simulink model "sphere_6SUR_mech"  (R2017a)
settings: Solver=FixedStepAuto  StartTime=0.0  StopTime=100  FixedStep=0.001  RelTol=1e-2  EnableMultiTasking=on
undefined symbols (not defined in the file): m, rad, s
libraries: mblibv1 x69, simulink x3, instrumentlib x1
(part 2 of 2)

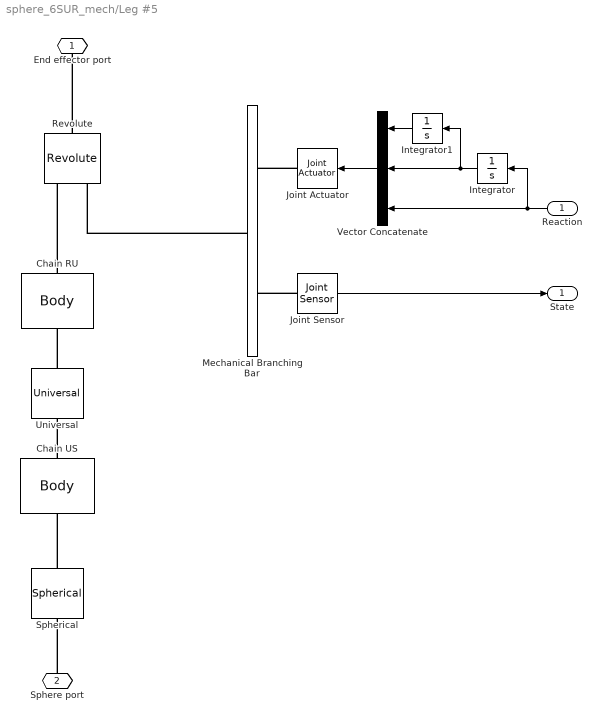
== system sphere_6SUR_mech/Leg #5 ==
  Reaction : Inport
  Chain RU : mblibv1/Bodies/Body  LConnTagsString=CS1  RConnTagsString=CS2  UpdateFromCAD=off  DialogClass=MechanicalBodyBlock  Mass=ru_mass  MassUnits=kg  InertiaUnits=kg*m^2  Inertia=zeros(3)  Shape=Cylinder  ShapeDims=[1 1]  ShapeUnits=m  ShapeUse=false  Density=1  DensityUnits=kg/m^3  DensityUse=false  GraphicsMode=CONVHULL  BodyColorSelMode=COLORPALETTE  BodyColor=[0 1 0]  AttachedToCS=CG  CG=Left$CG$(u_coord+r_coord)/2$World$World$m$[0 0 0]$Euler X-Y-Z$deg$World$false$none  WorkingFrames=Left$CS1$u_coord$World$World$m$[0 0 0]$Euler X-Y-Z$deg$World$true$none#Right$CS2$r_coord$World$World$m$[0 0 0]$Euler X-Y-Z$deg$World$true$none  CGPos=(u_coord+r_coord)/2  CGRot=[0 0 0]  CS0Pos=[]  CS0Rot=[]  CS1Pos=u_coord  CS1Rot=[0 0 0]  CS2Pos=r_coord  CS2Rot=[0 0 0]  CS3Pos=[]  CS3Rot=[]  CS4Pos=[]  CS4Rot=[]  CS5Pos=[]  CS5Rot=[]  CS6Pos=[]  CS6Rot=[]  CS7Pos=[]  CS7Rot=[]  CS8Pos=[]  CS8Rot=[]  CS9Pos=[]  CS9Rot=[]  CS10Pos=[]  CS10Rot=[]  CS11Pos=[]  CS11Rot=[]  CS12Pos=[]  CS12Rot=[]  CS13Pos=[]  CS13Rot=[]  CS14Pos=[]  CS14Rot=[]  CS15Pos=[]  CS15Rot=[]  CS16Pos=[]  CS16Rot=[]  CS17Pos=[]  CS17Rot=[]  CS18Pos=[]  CS18Rot=[]  CS19Pos=[]  CS19Rot=[]  CS20Pos=[]  CS20Rot=[]
      settings: SourceProductName=Simscape Multibody  SourceProductBaseCode=MS
  Chain US : mblibv1/Bodies/Body  LConnTagsString=CS1  RConnTagsString=CS2  UpdateFromCAD=off  DialogClass=MechanicalBodyBlock  Mass=us_mass  MassUnits=kg  InertiaUnits=kg*m^2  Inertia=zeros(3)  Shape=Cylinder  ShapeDims=[1 1]  ShapeUnits=m  ShapeUse=false  Density=1  DensityUnits=kg/m^3  DensityUse=false  GraphicsMode=CONVHULL  BodyColorSelMode=COLORPALETTE  BodyColor=[0 1 0]  AttachedToCS=CG  CG=Left$CG$(s_coord+u_coord)/2$World$World$m$[0 0 0]$Euler X-Y-Z$deg$World$false$none  WorkingFrames=Left$CS1$s_coord$World$World$m$[0 0 0]$Euler X-Y-Z$deg$World$true$none#Right$CS2$u_coord$World$World$m$[0 0 0]$Euler X-Y-Z$deg$World$true$none  CGPos=(s_coord+u_coord)/2  CGRot=[0 0 0]  CS0Pos=[]  CS0Rot=[]  CS1Pos=s_coord  CS1Rot=[0 0 0]  CS2Pos=u_coord  CS2Rot=[0 0 0]  CS3Pos=[]  CS3Rot=[]  CS4Pos=[]  CS4Rot=[]  CS5Pos=[]  CS5Rot=[]  CS6Pos=[]  CS6Rot=[]  CS7Pos=[]  CS7Rot=[]  CS8Pos=[]  CS8Rot=[]  CS9Pos=[]  CS9Rot=[]  CS10Pos=[]  CS10Rot=[]  CS11Pos=[]  CS11Rot=[]  CS12Pos=[]  CS12Rot=[]  CS13Pos=[]  CS13Rot=[]  CS14Pos=[]  CS14Rot=[]  CS15Pos=[]  CS15Rot=[]  CS16Pos=[]  CS16Rot=[]  CS17Pos=[]  CS17Rot=[]  CS18Pos=[]  CS18Rot=[]  CS19Pos=[]  CS19Rot=[]  CS20Pos=[]  CS20Rot=[]
      settings: SourceProductName=Simscape Multibody  SourceProductBaseCode=MS
  Integrator : Integrator
  Integrator1 : Integrator
  Joint Actuator : mblibv1/Sensors &  Actuators/Joint Actuator  UpdateFromCAD=off  PhysicalDomain=Mechanical  PortType=blob  ActuationStyle=Motion  AngleUnits=rad  ArcVelocityUnits=rad/s  ArcAccelerationUnits=rad/s^2  CoordPositionUnits=m  VelocityUnits=m/s  AccelerationUnits=m/s^2  ForceUnits=N  TorqueUnits=N*m  ActiveIO=on  Width=3  DialogClass=MechanicalActuatorBlock  Primitive=R1  ReferenceFrame=Absolute (World)
      settings: SourceProductName=Simscape Multibody  SourceProductBaseCode=MS
  Joint Sensor : mblibv1/Sensors &  Actuators/Joint Sensor  UpdateFromCAD=off  PhysicalDomain=Mechanical  PortType=blob  Muxed=on  Pose=off  Angle=on  AngleUnits=rad  ArcVelocity=on  ArcVelocityUnits=rad/s  ArcAcceleration=on  ArcAccelerationUnits=rad/s^2  CoordPosition=on  CoordPositionUnits=m  Velocity=on  VelocityUnits=m/s  Acceleration=on  AccelerationUnits=m/s^2  Quaternion=on  QuaternionDT=off  QuaternionDDT=off  QuaternionUnits=off  OutputVector=[1]  ActiveIO=on  Width=10  DialogClass=MechanicalSensorBlock  Primitive=R1  Force=on  ForceUnits=N  Torque=on  TorqueUnits=N*m  ReferenceFrame=Absolute (World)  ReactionSensedSide=Base  ReactionReferenceFrame=Local (Body CS)  ReactionForce=on  ReactionForceUnits=N  ReactionMoment=on  ReactionMomentUnits=N*m
      settings: SourceProductName=Simscape Multibody  SourceProductBaseCode=MS
  Mechanical Branching Bar : mblibv1/Utilities/Mechanical Branching Bar  LConnTagsString=_newl0  RConnTagsString=SA0|SA1  UpdateFromCAD=off  DialogClass=MechanicalBranchingBarBlock  NumSAPorts=2
      settings: SourceProductName=Simscape Multibody  SourceProductBaseCode=MS
  Revolute : mblibv1/Joints/Revolute  LConnTagsString=__newl0|SA1  RConnTagsString=__newr0  UpdateFromCAD=off  NumSAPorts=1  CutJoint=off  MarkAsCut=off  Primitives=prismatic  PrimitiveProps=R1$World$r_axis$revolute  DialogClass=JointBlock  R1Axis=r_axis
      settings: SourceProductName=Simscape Multibody  SourceProductBaseCode=MS
  Spherical : mblibv1/Joints/Spherical  LConnTagsString=__newl0  RConnTagsString=__newr0  UpdateFromCAD=off  NumSAPorts=0  CutJoint=off  MarkAsCut=off  Primitives=spherical  PrimitiveProps=S$WORLD$[0 0 0]$spherical  DialogClass=JointBlock  SAxis=[0 0 0]
      settings: SourceProductName=Simscape Multibody  SourceProductBaseCode=MS
  Universal : mblibv1/Joints/Universal  LConnTagsString=__newl0  RConnTagsString=__newr0  UpdateFromCAD=off  NumSAPorts=0  CutJoint=off  MarkAsCut=off  Primitives=prismatic  PrimitiveProps=R1$World$u_axis1$revolute#R2$World$u_axis2$revolute  DialogClass=JointBlock  R1Axis=u_axis1  R2Axis=u_axis2
      settings: SourceProductName=Simscape Multibody  SourceProductBaseCode=MS
  Vector Concatenate : Concatenate  NumInputs=3
  End effector port : PMIOPort  Port=1  Side=Right
  Sphere port : PMIOPort  Port=2  Side=Left
  State : Outport
  wires:
  Joint Sensor/1 -> State/1
  Vector Concatenate/1 -> Joint Actuator/1
  Reaction/1 -> Integrator/1, Vector Concatenate/3
  Integrator/1 -> Integrator1/1, Vector Concatenate/2
  Integrator1/1 -> Vector Concatenate/1
  connections:
  Revolute/RConn1 -- End effector port/RConn1
  Joint Actuator/RConn1 -- Mechanical Branching Bar/RConn1
  Chain RU/RConn1 -- Revolute/LConn1
  Mechanical Branching Bar/LConn1 -- Revolute/LConn2
  Joint Sensor/LConn1 -- Mechanical Branching Bar/RConn2
  Spherical/RConn1 -- Chain US/LConn1
  Universal/RConn1 -- Chain RU/LConn1
  Chain US/RConn1 -- Universal/LConn1
  Sphere port/RConn1 -- Spherical/LConn1

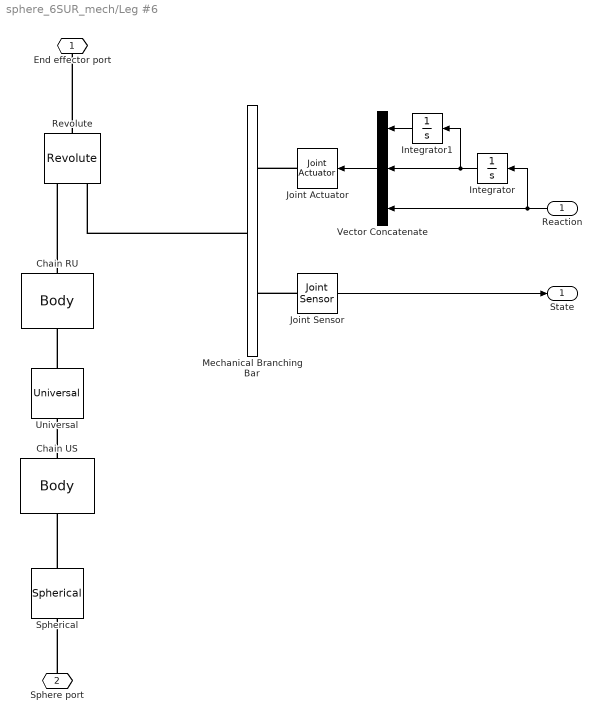
== system sphere_6SUR_mech/Leg #6 ==
  Reaction : Inport
  Chain RU : mblibv1/Bodies/Body  LConnTagsString=CS1  RConnTagsString=CS2  UpdateFromCAD=off  DialogClass=MechanicalBodyBlock  Mass=ru_mass  MassUnits=kg  InertiaUnits=kg*m^2  Inertia=zeros(3)  Shape=Cylinder  ShapeDims=[1 1]  ShapeUnits=m  ShapeUse=false  Density=1  DensityUnits=kg/m^3  DensityUse=false  GraphicsMode=CONVHULL  BodyColorSelMode=COLORPALETTE  BodyColor=[0 1 0]  AttachedToCS=CG  CG=Left$CG$(u_coord+r_coord)/2$World$World$m$[0 0 0]$Euler X-Y-Z$deg$World$false$none  WorkingFrames=Left$CS1$u_coord$World$World$m$[0 0 0]$Euler X-Y-Z$deg$World$true$none#Right$CS2$r_coord$World$World$m$[0 0 0]$Euler X-Y-Z$deg$World$true$none  CGPos=(u_coord+r_coord)/2  CGRot=[0 0 0]  CS0Pos=[]  CS0Rot=[]  CS1Pos=u_coord  CS1Rot=[0 0 0]  CS2Pos=r_coord  CS2Rot=[0 0 0]  CS3Pos=[]  CS3Rot=[]  CS4Pos=[]  CS4Rot=[]  CS5Pos=[]  CS5Rot=[]  CS6Pos=[]  CS6Rot=[]  CS7Pos=[]  CS7Rot=[]  CS8Pos=[]  CS8Rot=[]  CS9Pos=[]  CS9Rot=[]  CS10Pos=[]  CS10Rot=[]  CS11Pos=[]  CS11Rot=[]  CS12Pos=[]  CS12Rot=[]  CS13Pos=[]  CS13Rot=[]  CS14Pos=[]  CS14Rot=[]  CS15Pos=[]  CS15Rot=[]  CS16Pos=[]  CS16Rot=[]  CS17Pos=[]  CS17Rot=[]  CS18Pos=[]  CS18Rot=[]  CS19Pos=[]  CS19Rot=[]  CS20Pos=[]  CS20Rot=[]
      settings: SourceProductName=Simscape Multibody  SourceProductBaseCode=MS
  Chain US : mblibv1/Bodies/Body  LConnTagsString=CS1  RConnTagsString=CS2  UpdateFromCAD=off  DialogClass=MechanicalBodyBlock  Mass=us_mass  MassUnits=kg  InertiaUnits=kg*m^2  Inertia=zeros(3)  Shape=Cylinder  ShapeDims=[1 1]  ShapeUnits=m  ShapeUse=false  Density=1  DensityUnits=kg/m^3  DensityUse=false  GraphicsMode=CONVHULL  BodyColorSelMode=COLORPALETTE  BodyColor=[0 1 0]  AttachedToCS=CG  CG=Left$CG$(s_coord+u_coord)/2$World$World$m$[0 0 0]$Euler X-Y-Z$deg$World$false$none  WorkingFrames=Left$CS1$s_coord$World$World$m$[0 0 0]$Euler X-Y-Z$deg$World$true$none#Right$CS2$u_coord$World$World$m$[0 0 0]$Euler X-Y-Z$deg$World$true$none  CGPos=(s_coord+u_coord)/2  CGRot=[0 0 0]  CS0Pos=[]  CS0Rot=[]  CS1Pos=s_coord  CS1Rot=[0 0 0]  CS2Pos=u_coord  CS2Rot=[0 0 0]  CS3Pos=[]  CS3Rot=[]  CS4Pos=[]  CS4Rot=[]  CS5Pos=[]  CS5Rot=[]  CS6Pos=[]  CS6Rot=[]  CS7Pos=[]  CS7Rot=[]  CS8Pos=[]  CS8Rot=[]  CS9Pos=[]  CS9Rot=[]  CS10Pos=[]  CS10Rot=[]  CS11Pos=[]  CS11Rot=[]  CS12Pos=[]  CS12Rot=[]  CS13Pos=[]  CS13Rot=[]  CS14Pos=[]  CS14Rot=[]  CS15Pos=[]  CS15Rot=[]  CS16Pos=[]  CS16Rot=[]  CS17Pos=[]  CS17Rot=[]  CS18Pos=[]  CS18Rot=[]  CS19Pos=[]  CS19Rot=[]  CS20Pos=[]  CS20Rot=[]
      settings: SourceProductName=Simscape Multibody  SourceProductBaseCode=MS
  Integrator : Integrator
  Integrator1 : Integrator
  Joint Actuator : mblibv1/Sensors &  Actuators/Joint Actuator  UpdateFromCAD=off  PhysicalDomain=Mechanical  PortType=blob  ActuationStyle=Motion  AngleUnits=rad  ArcVelocityUnits=rad/s  ArcAccelerationUnits=rad/s^2  CoordPositionUnits=m  VelocityUnits=m/s  AccelerationUnits=m/s^2  ForceUnits=N  TorqueUnits=N*m  ActiveIO=on  Width=3  DialogClass=MechanicalActuatorBlock  Primitive=R1  ReferenceFrame=Absolute (World)
      settings: SourceProductName=Simscape Multibody  SourceProductBaseCode=MS
  Joint Sensor : mblibv1/Sensors &  Actuators/Joint Sensor  UpdateFromCAD=off  PhysicalDomain=Mechanical  PortType=blob  Muxed=on  Pose=off  Angle=on  AngleUnits=rad  ArcVelocity=on  ArcVelocityUnits=rad/s  ArcAcceleration=on  ArcAccelerationUnits=rad/s^2  CoordPosition=on  CoordPositionUnits=m  Velocity=on  VelocityUnits=m/s  Acceleration=on  AccelerationUnits=m/s^2  Quaternion=on  QuaternionDT=off  QuaternionDDT=off  QuaternionUnits=off  OutputVector=[1]  ActiveIO=on  Width=10  DialogClass=MechanicalSensorBlock  Primitive=R1  Force=on  ForceUnits=N  Torque=on  TorqueUnits=N*m  ReferenceFrame=Absolute (World)  ReactionSensedSide=Base  ReactionReferenceFrame=Local (Body CS)  ReactionForce=on  ReactionForceUnits=N  ReactionMoment=on  ReactionMomentUnits=N*m
      settings: SourceProductName=Simscape Multibody  SourceProductBaseCode=MS
  Mechanical Branching Bar : mblibv1/Utilities/Mechanical Branching Bar  LConnTagsString=_newl0  RConnTagsString=SA0|SA1  UpdateFromCAD=off  DialogClass=MechanicalBranchingBarBlock  NumSAPorts=2
      settings: SourceProductName=Simscape Multibody  SourceProductBaseCode=MS
  Revolute : mblibv1/Joints/Revolute  LConnTagsString=__newl0|SA1  RConnTagsString=__newr0  UpdateFromCAD=off  NumSAPorts=1  CutJoint=off  MarkAsCut=off  Primitives=prismatic  PrimitiveProps=R1$World$r_axis$revolute  DialogClass=JointBlock  R1Axis=r_axis
      settings: SourceProductName=Simscape Multibody  SourceProductBaseCode=MS
  Spherical : mblibv1/Joints/Spherical  LConnTagsString=__newl0  RConnTagsString=__newr0  UpdateFromCAD=off  NumSAPorts=0  CutJoint=off  MarkAsCut=off  Primitives=spherical  PrimitiveProps=S$WORLD$[0 0 0]$spherical  DialogClass=JointBlock  SAxis=[0 0 0]
      settings: SourceProductName=Simscape Multibody  SourceProductBaseCode=MS
  Universal : mblibv1/Joints/Universal  LConnTagsString=__newl0  RConnTagsString=__newr0  UpdateFromCAD=off  NumSAPorts=0  CutJoint=off  MarkAsCut=off  Primitives=prismatic  PrimitiveProps=R1$World$u_axis1$revolute#R2$World$u_axis2$revolute  DialogClass=JointBlock  R1Axis=u_axis1  R2Axis=u_axis2
      settings: SourceProductName=Simscape Multibody  SourceProductBaseCode=MS
  Vector Concatenate : Concatenate  NumInputs=3
  End effector port : PMIOPort  Port=1  Side=Right
  Sphere port : PMIOPort  Port=2  Side=Left
  State : Outport
  wires:
  Joint Sensor/1 -> State/1
  Vector Concatenate/1 -> Joint Actuator/1
  Reaction/1 -> Integrator/1, Vector Concatenate/3
  Integrator/1 -> Integrator1/1, Vector Concatenate/2
  Integrator1/1 -> Vector Concatenate/1
  connections:
  Revolute/RConn1 -- End effector port/RConn1
  Joint Actuator/RConn1 -- Mechanical Branching Bar/RConn1
  Chain RU/RConn1 -- Revolute/LConn1
  Mechanical Branching Bar/LConn1 -- Revolute/LConn2
  Joint Sensor/LConn1 -- Mechanical Branching Bar/RConn2
  Spherical/RConn1 -- Chain US/LConn1
  Universal/RConn1 -- Chain RU/LConn1
  Chain US/RConn1 -- Universal/LConn1
  Sphere port/RConn1 -- Spherical/LConn1

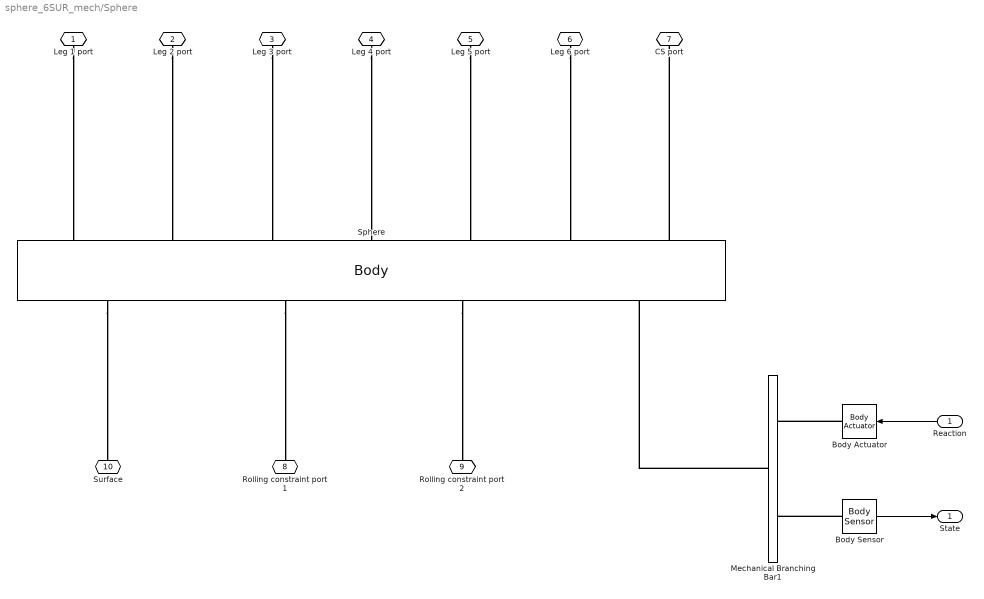
== system sphere_6SUR_mech/Sphere ==
  Reaction : Inport  OutDataTypeStr=double
  Body Actuator : mblibv1/Sensors &  Actuators/Body Actuator  UpdateFromCAD=off  PhysicalDomain=Mechanical  PortType=blob  ActuationStyle=Force  AngleUnits=deg  ArcVelocityUnits=deg/s  ArcAccelerationUnits=deg/s^2  CoordPositionUnits=m  VelocityUnits=m/s  AccelerationUnits=m/s^2  ForceUnits=N  TorqueUnits=N*m  ActiveIO=on  Width=6  DialogClass=MechanicalActuatorBlock  ReferenceFrame=Absolute (World)  Angle=off  CoordPosition=on  Force=on  Torque=on
      settings: SourceProductName=Simscape Multibody  SourceProductBaseCode=MS
  Body Sensor : mblibv1/Sensors &  Actuators/Body Sensor  UpdateFromCAD=off  PhysicalDomain=Mechanical  PortType=blob  Muxed=on  Pose=on  Angle=on  AngleUnits=deg  ArcVelocity=on  ArcVelocityUnits=rad/s  ArcAcceleration=on  ArcAccelerationUnits=rad/s^2  CoordPosition=on  CoordPositionUnits=m  Velocity=on  VelocityUnits=m/s  Acceleration=on  AccelerationUnits=m/s^2  Quaternion=on  QuaternionDT=off  QuaternionDDT=off  QuaternionUnits=off  OutputVector=[1]  ActiveIO=on  Width=24  DialogClass=MechanicalSensorBlock  ReferenceFrame=Absolute (World)
      settings: SourceProductName=Simscape Multibody  SourceProductBaseCode=MS
  Mechanical Branching Bar1 : mblibv1/Utilities/Mechanical Branching Bar  LConnTagsString=_newl0  RConnTagsString=SA0|SA1  UpdateFromCAD=off  DialogClass=MechanicalBranchingBarBlock  NumSAPorts=2
      settings: SourceProductName=Simscape Multibody  SourceProductBaseCode=MS
  Sphere : mblibv1/Bodies/Body  LConnTagsString=CG|CS8|CS9|CS10  RConnTagsString=CS1|CS2|CS3|CS4|CS5|CS6|CS7  UpdateFromCAD=off  DialogClass=MechanicalBodyBlock  Mass=sphere_mass  MassUnits=kg  InertiaUnits=kg*m^2  Inertia=sphere_inertia_coef*sphere_mass*sphere_radius^2*eye(3)  Shape=Cylinder  ShapeDims=[1 1]  ShapeUnits=m  ShapeUse=false  Density=1  DensityUnits=kg/m^3  DensityUse=false  GraphicsMode=EQELLIPSE  BodyColorSelMode=COLORPALETTE  BodyColor=[0 0 0]  AttachedToCS=CG  CG=Left$CG$[0; 0; 0]$World$World$m$[0 0 0]$Euler X-Y-Z$deg$World$true$none  WorkingFrames=Right$CS1$[0; 0; 0]$Adjoining$Adjoining$m$[0 0 0]$Euler X-Y-Z$deg$CG$true$none#Right$CS2$[0; 0; 0]$Adjoining$Adjoining$m$[0 0 0]$Euler X-Y-Z$deg$CG$true$none#Right$CS3$[0; 0; 0]$Adjoining$Adjoining$m$[0 0 0]$Euler X-Y-Z$deg$CG$true$none#Right$CS4$[0; 0; 0]$Adjoining$Adjoining$m$[0 0 0]$Euler X-Y-Z$deg$CG$true$none#Right$CS5$[0; 0; 0]$Adjoining$Adjoining$m$[0 0 0]$Euler X-Y-Z$deg$CG$true$none#Right$CS6$[0; 0; 0]$Adjoining$Adjoining$m$[0 0 0]$Euler X-Y-Z$deg$CG$true$none#Right$CS7$[0; 0; 0]$World$World$m$[0 0 0]$Euler X-Y-Z$deg$CG$true$none#Left$CS8$[0; 0; 0]$World$World$m$[0 0 0]$Euler X-Y-Z$deg$CG$true$none#Left$CS9$[0; 0; 0]$World$World$m$[0 0 0]$Euler X-Y-Z$deg$CG$true$none#Left$CS10$[0; 0; 0]$World$World$m$[0 0 0]$Euler X-Y-Z$deg$CG$true$none  CGPos=[0; 0; 0]  CGRot=[0 0 0]  CS0Pos=[]  CS0Rot=[]  CS1Pos=[0; 0; 0]  CS1Rot=[0 0 0]  CS2Pos=[0; 0; 0]  CS2Rot=[0 0 0]  CS3Pos=[0; 0; 0]  CS3Rot=[0 0 0]  CS4Pos=[0; 0; 0]  CS4Rot=[0 0 0]  CS5Pos=[0; 0; 0]  CS5Rot=[0 0 0]  CS6Pos=[0; 0; 0]  CS6Rot=[0 0 0]  CS7Pos=[0; 0; 0]  CS7Rot=[0 0 0]  CS8Pos=[0; 0; 0]  CS8Rot=[0 0 0]  CS9Pos=[0; 0; 0]  CS9Rot=[0 0 0]  CS10Pos=[0; 0; 0]  CS10Rot=[0 0 0]  CS11Pos=[]  CS11Rot=[]  CS12Pos=[]  CS12Rot=[]  CS13Pos=[]  CS13Rot=[]  CS14Pos=[]  CS14Rot=[]  CS15Pos=[]  CS15Rot=[]  CS16Pos=[]  CS16Rot=[]  CS17Pos=[]  CS17Rot=[]  CS18Pos=[]  CS18Rot=[]  CS19Pos=[]  CS19Rot=[]  CS20Pos=[]  CS20Rot=[]
      settings: SourceProductName=Simscape Multibody  SourceProductBaseCode=MS
  Leg 1 port : PMIOPort  Port=1  Side=Right
  Leg 2 port : PMIOPort  Port=2  Side=Right
  Leg 3 port : PMIOPort  Port=3  Side=Right
  Leg 4 port : PMIOPort  Port=4  Side=Right
  Leg 5 port : PMIOPort  Port=5  Side=Right
  Leg 6 port : PMIOPort  Port=6  Side=Right
  CS port : PMIOPort  Port=7  Side=Right
  Rolling constraint port 1 : PMIOPort  Port=8  Side=Left
  Rolling constraint port 2 : PMIOPort  Port=9  Side=Left
  Surface : PMIOPort  Port=10  Side=Left
  State : Outport  OutDataTypeStr=double
  wires:
  Reaction/1 -> Body Actuator/1
  Body Sensor/1 -> State/1
  connections:
  Sphere/LConn3 -- Rolling constraint port 2/RConn1
  Sphere/LConn2 -- Rolling constraint port 1/RConn1
  Sphere/LConn1 -- Surface/RConn1
  Sphere/RConn7 -- CS port/RConn1
  Leg 5 port/RConn1 -- Sphere/RConn5
  Leg 6 port/RConn1 -- Sphere/RConn6
  Leg 4 port/RConn1 -- Sphere/RConn4
  Leg 2 port/RConn1 -- Sphere/RConn2
  Leg 3 port/RConn1 -- Sphere/RConn3
  Leg 1 port/RConn1 -- Sphere/RConn1
  Mechanical Branching Bar1/LConn1 -- Sphere/LConn4
  Body Sensor/LConn1 -- Mechanical Branching Bar1/RConn2
  Body Actuator/RConn1 -- Mechanical Branching Bar1/RConn1

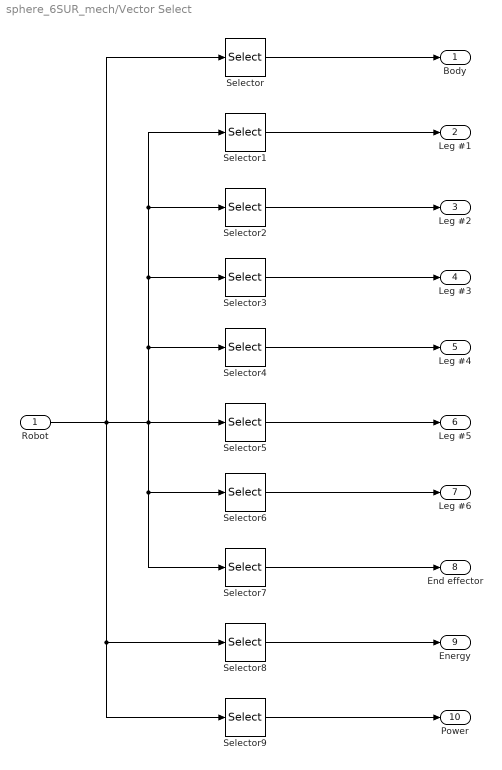
== system sphere_6SUR_mech/Vector Select ==
  Robot : Inport
  Selector : Selector  IndexOptions=Starting index (dialog)  Indices=1  OutputSizes=6
  Selector1 : Selector  IndexOptions=Starting index (dialog)  Indices=7  OutputSizes=1
  Selector2 : Selector  IndexOptions=Starting index (dialog)  Indices=8  OutputSizes=1
  Selector3 : Selector  IndexOptions=Starting index (dialog)  Indices=9  OutputSizes=1
  Selector4 : Selector  IndexOptions=Starting index (dialog)  Indices=10  OutputSizes=1
  Selector5 : Selector  IndexOptions=Starting index (dialog)  Indices=11  OutputSizes=1
  Selector6 : Selector  IndexOptions=Starting index (dialog)  Indices=12  OutputSizes=1
  Selector7 : Selector  IndexOptions=Starting index (dialog)  Indices=13  OutputSizes=6
  Selector8 : Selector  IndexOptions=Starting index (dialog)  Indices=19  OutputSizes=1
  Selector9 : Selector  IndexOptions=Starting index (dialog)  Indices=20  OutputSizes=1
  Body : Outport
  Leg #1 : Outport  Port=2
  Leg #2 : Outport  Port=3
  Leg #3 : Outport  Port=4
  Leg #4 : Outport  Port=5
  Leg #5 : Outport  Port=6
  Leg #6 : Outport  Port=7
  End effector : Outport  Port=8
  Energy : Outport  Port=9
  Power : Outport  Port=10
  wires:
  Selector7/1 -> End effector/1
  Selector2/1 -> Leg #2/1
  Selector1/1 -> Leg #1/1
  Selector3/1 -> Leg #3/1
  Selector/1 -> Body/1
  Robot/1 -> Selector1/1, Selector2/1, Selector3/1, Selector4/1, Selector5/1, Selector6/1, Selector7/1, Selector/1, Selector8/1, Selector9/1
  Selector8/1 -> Energy/1
  Selector9/1 -> Power/1
  Selector5/1 -> Leg #5/1
  Selector4/1 -> Leg #4/1
  Selector6/1 -> Leg #6/1

== system sphere_6SUR_mech/Environment/Plane ==
  Constraint Point : mblibv1/Bodies/Body  LConnTagsString=CG  RConnTagsString=CS5  UpdateFromCAD=off  DialogClass=MechanicalBodyBlock  Mass=0  MassUnits=kg  InertiaUnits=kg*m^2  Inertia=zeros(3)  Shape=Cylinder  ShapeDims=[1 1]  ShapeUnits=m  ShapeUse=false  Density=1  DensityUnits=kg/m^3  DensityUse=false  GraphicsMode=CONVHULL  BodyColorSelMode=COLORPALETTE  BodyColor=[0.23137 0.44314 0.33725]  AttachedToCS=CG  CG=Left$CG$[0 0 0]$WORLD$WORLD$m$[0 0 0]$Euler X-Y-Z$deg$WORLD$true$none  WorkingFrames=Right$CS5$[0 0 0]$Adjoining$Adjoining$m$[0 0 0]$Euler X-Y-Z$deg$WORLD$true$none  CGPos=[0 0 0]  CGRot=[0 0 0]  CS0Pos=[]  CS0Rot=[]  CS1Pos=[]  CS1Rot=[]  CS2Pos=[]  CS2Rot=[]  CS3Pos=[]  CS3Rot=[]  CS4Pos=[]  CS4Rot=[]  CS5Pos=[0 0 0]  CS5Rot=[0 0 0]  CS6Pos=[]  CS6Rot=[]  CS7Pos=[]  CS7Rot=[]  CS8Pos=[]  CS8Rot=[]  CS9Pos=[]  CS9Rot=[]  CS10Pos=[]  CS10Rot=[]  CS11Pos=[]  CS11Rot=[]  CS12Pos=[]  CS12Rot=[]  CS13Pos=[]  CS13Rot=[]  CS14Pos=[]  CS14Rot=[]  CS15Pos=[]  CS15Rot=[]  CS16Pos=[]  CS16Rot=[]  CS17Pos=[]  CS17Rot=[]  CS18Pos=[]  CS18Rot=[]  CS19Pos=[]  CS19Rot=[]  CS20Pos=[]  CS20Rot=[]
      settings: SourceProductName=Simscape Multibody  SourceProductBaseCode=MS
  Ground : mblibv1/Bodies/Ground  UpdateFromCAD=off  LeftPortType=env  RightPortType=workingframe  PhysicalDomain=Mechanical  DialogClass=GroundBlock  CoordPosition=[0 0 -sphere_radius]  CoordPositionUnits=m  StateVectorMgrId=0  MachineId=[1 0]  ShowEnvPort=on  ParameterChecksum=[1237703070, 1025381231, 1062509031, 856793799]  TopologyChecksum=[360264477, 2755086963, 1397278036, 1502798817]
      settings: SourceProductName=Simscape Multibody  SourceProductBaseCode=MS
  Machine Environment : mblibv1/Bodies/Machine Environment  Tag=Factory ground  PortType=env  PhysicalDomain=Mechanical  DialogTemplateClass=MECH.MachineEnvironment  SyncWhenCopied=off  Gravity=[0 0 -9.81]  GravityUnits=m/s^2  GravityAsSignal=off  Dimensionality=3D Only  AnalysisType=Forward dynamics  LinearAssemblyTolerance=1e-3  LinearAssemblyToleranceUnits=m  AngularAssemblyTolerance=1e-3  AngularAssemblyToleranceUnits=rad  ConstraintSolverType=Stabilizing  ConstraintRelTolerance=1e-4  ConstraintAbsTolerance=1e-4  UseRobustSingularityHandling=off  RedundancyAnalysisToleranceType=Automatically select tolerance  RedundancyAnalysisTolerance=1e-14  StatePerturbationType=Fixed  PerturbationSize=1e-5  VisualizeMachine=on  BodyVisualizationType=Use model default body geometries  BodyColorSelMode=Use model default  DefaultBodyColor=[1 0 0]
      settings: SourceProductName=Simscape Multibody  SourceProductBaseCode=MS
  Plane : mblibv1/Bodies/Body  LConnTagsString=CG  RConnTagsString=CS1  UpdateFromCAD=off  DialogClass=MechanicalBodyBlock  Mass=1  MassUnits=kg  InertiaUnits=kg*m^2  Inertia=(1/12)*[400 0 0;0 400 0;0 0 800]  Shape=Cylinder  ShapeDims=[1 1]  ShapeUnits=m  ShapeUse=false  Density=1  DensityUnits=kg/m^3  DensityUse=false  GraphicsMode=CONVHULL  BodyColorSelMode=COLORPALETTE  BodyColor=[0.23137 0.44314 0.33725]  AttachedToCS=CG  CG=Left$CG$[0 0 0]$CS1$CS1$m$[0 0 0]$Euler X-Y-Z$deg$WORLD$true$none  WorkingFrames=Right$CS1$[0 0 0]$Adjoining$Adjoining$m$[0 0 0]$Euler X-Y-Z$deg$WORLD$true$none#Right$CS2$[width width 0]$CG$CG$m$[0 0 0]$Euler X-Y-Z$deg$WORLD$false$none#Right$CS3$[width -width 0]$CG$CG$m$[0 0 0]$Euler X-Y-Z$deg$WORLD$false$none#Right$CS4$[-width width 0]$CG$CG$m$[0 0 0]$Euler X-Y-Z$deg$WORLD$false$none#Right$CS5$[-width -width 0]$CG$CG$m$[0 0 0]$Euler X-Y-Z$deg$WORLD$false$none  CGPos=[0 0 0]  CGRot=[0 0 0]  CS0Pos=[]  CS0Rot=[]  CS1Pos=[0 0 0]  CS1Rot=[0 0 0]  CS2Pos=[width width 0]  CS2Rot=[0 0 0]  CS3Pos=[width -width 0]  CS3Rot=[0 0 0]  CS4Pos=[-width width 0]  CS4Rot=[0 0 0]  CS5Pos=[-width -width 0]  CS5Rot=[0 0 0]  CS6Pos=[]  CS6Rot=[]  CS7Pos=[]  CS7Rot=[]  CS8Pos=[]  CS8Rot=[]  CS9Pos=[]  CS9Rot=[]  CS10Pos=[]  CS10Rot=[]  CS11Pos=[]  CS11Rot=[]  CS12Pos=[]  CS12Rot=[]  CS13Pos=[]  CS13Rot=[]  CS14Pos=[]  CS14Rot=[]  CS15Pos=[]  CS15Rot=[]  CS16Pos=[]  CS16Rot=[]  CS17Pos=[]  CS17Rot=[]  CS18Pos=[]  CS18Rot=[]  CS19Pos=[]  CS19Rot=[]  CS20Pos=[]  CS20Rot=[]
      settings: SourceProductName=Simscape Multibody  SourceProductBaseCode=MS
  Weld : mblibv1/Joints/Weld  LConnTagsString=__newl0  RConnTagsString=__newr0  UpdateFromCAD=off  NumSAPorts=0  CutJoint=off  MarkAsCut=off  Primitives=weld  PrimitiveProps=W$WORLD$[0 0 0]$weld  DialogClass=JointBlock  WAxis=[0 0 0]
      settings: SourceProductName=Simscape Multibody  SourceProductBaseCode=MS
  Weld1 : mblibv1/Joints/Weld  LConnTagsString=__newl0  RConnTagsString=__newr0  UpdateFromCAD=off  NumSAPorts=0  CutJoint=off  MarkAsCut=off  Primitives=weld  PrimitiveProps=W$WORLD$[0 0 0]$weld  DialogClass=JointBlock  WAxis=[0 0 0]
      settings: SourceProductName=Simscape Multibody  SourceProductBaseCode=MS
  Point : PMIOPort  Port=1  Side=Left
  connections:
  Weld1/RConn1 -- Constraint Point/RConn1
  Machine Environment/RConn1 -- Ground/LConn1
  Ground/RConn1 -- Weld/LConn1
  Plane/LConn1 -- Weld1/LConn1
  Plane/RConn1 -- Weld/RConn1
  Point/RConn1 -- Constraint Point/LConn1

== system sphere_6SUR_mech/Environment/Rolling constraint ==
  note: vel_x = + omega_y
      | vel_y = - omega_x
  First rolling constraint : mblibv1/Constraints &  Drivers/Velocity Driver  LConnTagsString=__newl0  RConnTagsString=__newr0  UpdateFromCAD=off  DialogClass=ConstantVelocityConstraint  NumSAPorts=0  Unit_V=m/s  Unit_Omega=rad/s  Coef_V_Base=[1 0 0]  Csys_V_Base=World  Coef_Omega_Base=[0 -1 0]  Csys_Omega_Base=World  Coef_V_Follower=[0 0 0]  Csys_V_Follower=World  Coef_Omega_Follower=[0 0 0]  Csys_Omega_Follower=World
      settings: SourceProductName=Simscape Multibody  SourceProductBaseCode=MS
  Ground1 : mblibv1/Bodies/Ground  UpdateFromCAD=off  LeftPortType=env  RightPortType=workingframe  PhysicalDomain=Mechanical  DialogClass=GroundBlock  CoordPosition=[0 0 0]  CoordPositionUnits=m  StateVectorMgrId=-1  MachineId=[0 0]  ShowEnvPort=off  ParameterChecksum=[0 0 0 0]  TopologyChecksum=[0 0 0 0]
      settings: SourceProductName=Simscape Multibody  SourceProductBaseCode=MS
  Ground2 : mblibv1/Bodies/Ground  UpdateFromCAD=off  LeftPortType=env  RightPortType=workingframe  PhysicalDomain=Mechanical  DialogClass=GroundBlock  CoordPosition=[0 0 0]  CoordPositionUnits=m  StateVectorMgrId=-1  MachineId=[0 0]  ShowEnvPort=off  ParameterChecksum=[0 0 0 0]  TopologyChecksum=[0 0 0 0]
      settings: SourceProductName=Simscape Multibody  SourceProductBaseCode=MS
  Second rolling constraint : mblibv1/Constraints &  Drivers/Velocity Driver  LConnTagsString=__newl0  RConnTagsString=__newr0  UpdateFromCAD=off  DialogClass=ConstantVelocityConstraint  NumSAPorts=0  Unit_V=m/s  Unit_Omega=rad/s  Coef_V_Base=[0 1 0]  Csys_V_Base=World  Coef_Omega_Base=[1 0 0]  Csys_Omega_Base=World  Coef_V_Follower=[0 0 0]  Csys_V_Follower=World  Coef_Omega_Follower=[0 0 0]  Csys_Omega_Follower=World
      settings: SourceProductName=Simscape Multibody  SourceProductBaseCode=MS
  Constraint 1 : PMIOPort  Port=1  Side=Left
  Constraint 2 : PMIOPort  Port=2  Side=Left
  connections:
  First rolling constraint/RConn1 -- Ground1/RConn1
  Second rolling constraint/RConn1 -- Ground2/RConn1
  Constraint 2/RConn1 -- Second rolling constraint/LConn1
  Constraint 1/RConn1 -- First rolling constraint/LConn1
